simulink model "final_mppt_Algorithm_simuation_01"  (R2016a)
settings: Solver=VariableStepAuto  StartTime=0.0  StopTime=10.0  RelTol=1e-3
undefined symbols (not defined in the file or in its folder): sigbuilder_block
libraries: powerlib x12, simulink x2, powerlib_meascontrol x1
settings Model: Creator=Dell  LastModifiedBy=Dell

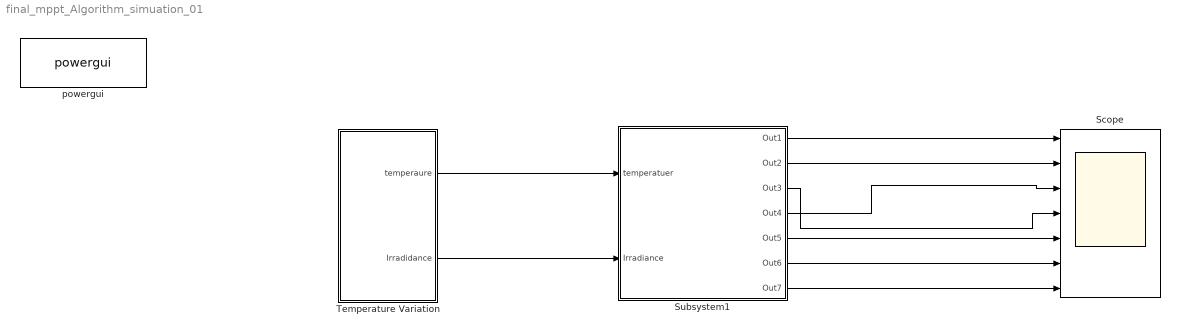
== system final_mppt_Algorithm_simuation_01 ==
  "Scope " : Scope  NumInputPorts=7
  Subsystem1 : Subsystem
  "Temperature Variation " : Subsystem  TreatAsAtomicUnit=on  VariantControl=Temperature
  powergui : powerlib/powergui  Priority=1  SimulationMode=Discrete  SolverType=Tustin  SampleTime=1e-6  frequency=60  SPID=off  DisableSnubberDevices=off  DisableRonSwitches=off  DisableVfSwitches=off  SwTol=0  DisplayEquations=off  Interpol=off  ExternalGateDelay=off  methode=off  Ts=0  FunctionMessages=off  echomessages=off  HookPort=off  EnableUseOfTLC=off  x0status=blocks  frequencyindice=0  Pbase=100e6  ErrMax=1e-4  Iterations=50  UnitsV=kV  UnitsW=MW  buscounter=0  RestoreLinks=warning  ResistiveCurrentMeasurement=off  Frange=[0:2:500]  Ylog=off  Xlog=on  ShowGrid=off  save=off  variable=ZData  structure=0  ZoomFFT=off  StartTime=0.0  cycles=1  DisplayStyle=1  fundamental=60  FreqAxis=off  MaxFrequency=1000  frequencyindicesteady=1  RmsSteady=1  display=off
  wires:
  "Temperature Variation "/1(temperaure) -> Subsystem1/1(temperatuer)
  "Temperature Variation "/2("Irradidance ") -> Subsystem1/2(Irradiance)
  Subsystem1/1(Out1) -> "Scope "/1
  Subsystem1/2(Out2) -> "Scope "/2
  Subsystem1/3(Out3) -> "Scope "/4
  Subsystem1/4(Out4) -> "Scope "/3
  Subsystem1/5(Out5) -> "Scope "/5
  Subsystem1/6(Out6) -> "Scope "/6
  Subsystem1/7(Out7) -> "Scope "/7

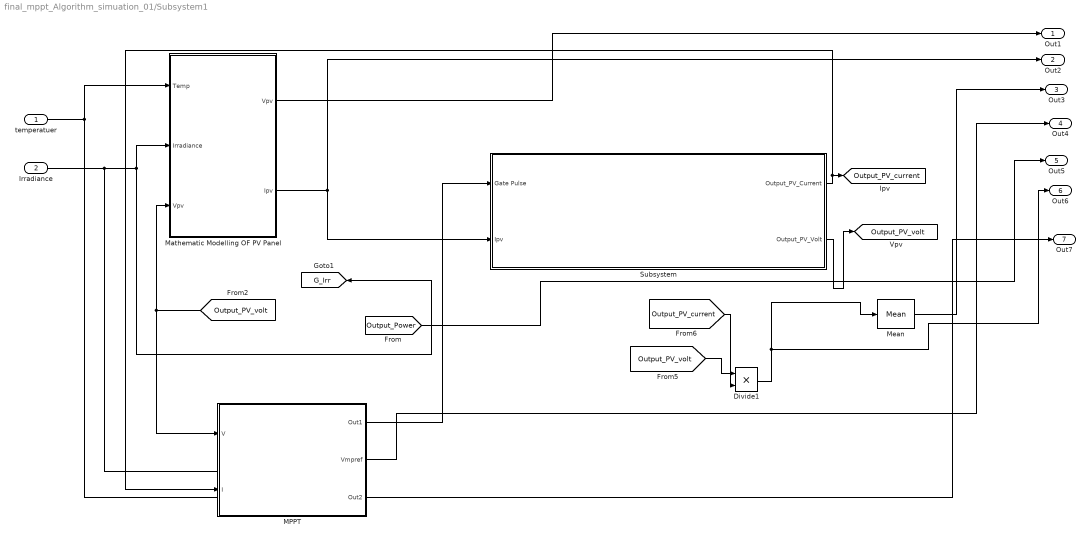
== system final_mppt_Algorithm_simuation_01/Subsystem1 ==
  temperatuer : Inport
  Irradiance : Inport  Port=2
  Divide1 : Product  Inputs=**
  MPPT : Subsystem
  Mathematic Modelling OF PV Panel : Subsystem
      mask Display:
      | plot([0.3 0.4],[0.4 0.8]);
      | plot([0.4 0.5],[0.4 0.8]);
      | plot([0.5 0.6],[0.4 0.8]);
      | plot([0.6 0.7],[0.4 0.8]);
      | plot([0.3 0.6],[0.4 0.4]);
      | plot([0.325 0.625],[0.5 0.5]);
      | plot([0.35 0.65],[0.6 0.6]);
      | plot([0.375 0.675],[0.7 0.7]);
      | plot([0.4 0.7],[0.8 0.8]);
      | text(0.52,0.75,'PV module (V)','horizontalAlignment', 'center');
  Mean : powerlib_meascontrol/Measurements/Mean  Freq=60  Vinit=0  Ts=0
  Subsystem : Subsystem
  Out1 : Outport
  Out2 : Outport  Port=2
  Out3 : Outport  Port=3
  Out4 : Outport  Port=4
  Out5 : Outport  Port=5
  Out6 : Outport  Port=6
  Out7 : Outport  Port=7
  tag scope: G_Irr=global, Output_PV_current=global, Output_PV_volt=global
  wires:
  [Output_PV_volt] -> Mathematic Modelling OF PV Panel/3(Vpv), MPPT/1(V)
  Irradiance/1 -> [G_Irr], Mathematic Modelling OF PV Panel/2(Irradiance)
  MPPT/2(Vmpref) -> Out4/1
  Mean/1 -> Out3/1
  Mathematic Modelling OF PV Panel/2(Ipv) -> Subsystem/2(Ipv), Out2/1
  MPPT/1(Out1) -> Subsystem/1(Gate Pulse)
  MPPT/3(Out2) -> Out7/1
  Mathematic Modelling OF PV Panel/1("Vpv ") -> Out1/1
  Divide1/1 -> Out6/1, Mean/1
  temperatuer/1 -> Mathematic Modelling OF PV Panel/1(Temp)
  Subsystem/1(Output_PV_Current) -> MPPT/2(I), [Output_PV_current]
  [Output_PV_volt] -> Divide1/1
  [Output_Power] -> Out5/1
  Subsystem/2(Output_PV_Volt) -> [Output_PV_volt]
  [Output_PV_current] -> Divide1/2

== system final_mppt_Algorithm_simuation_01/Temperature Variation  ==
  IRRADIANCE : Subsystem  Tag=STV Subsys  LoadFcn=sigbuilder_block('load');  StartFcn=sigbuilder_block('start');  StopFcn=sigbuilder_block('stop');  ClipboardFcn=sigbuilder_block('clipboard');  mask(Sigbuilder block){}
      mask help: Simulink:masks:SigbuilderBlock_MD
      mask init:
      | if ~strcmp(get_param(bdroot(gcbh),'SimulationStatus'),'stopped') tuvar = sigbuilder_block('maskInit'); end
      settings: CopyFcn=sigbuilder_block('copy');  DeleteFcn=sigbuilder_block('delete');  ModelCloseFcn=sigbuilder_block('modelClose');  PreSaveFcn=sigbuilder_block('preSave');  PauseFcn=sigbuilder_block('pause');  ContinueFcn=sigbuilder_block('continue');  NameChangeFcn=sigbuilder_block('namechange');  OpenFcn=sigbuilder_block('open',[6 28.2 1012.8 484.8 ]);  CloseFcn=sigbuilder_block('close');
      mask Display: plot(0, 0, 100, 100,[2, 2, 32, 32, 2], [68, 8, 8, 68, 68],[32, 2], [38, 38], [32, 19, 2],[53, 60, 44], [32, 17, 17, 2],[16, 16, 31, 31]);txt = getActiveGroup(gcbh);text(2, 100, txt,'verticalAlignment', 'top');
  TEMP : Subsystem  Tag=STV Subsys  LoadFcn=sigbuilder_block('load');  StartFcn=sigbuilder_block('start');  StopFcn=sigbuilder_block('stop');  ClipboardFcn=sigbuilder_block('clipboard');  mask(Sigbuilder block){}
      mask help: Simulink:masks:SigbuilderBlock_MD
      mask init:
      | if ~strcmp(get_param(bdroot(gcbh),'SimulationStatus'),'stopped') tuvar = sigbuilder_block('maskInit'); end
      settings: CopyFcn=sigbuilder_block('copy');  DeleteFcn=sigbuilder_block('delete');  ModelCloseFcn=sigbuilder_block('modelClose');  PreSaveFcn=sigbuilder_block('preSave');  PauseFcn=sigbuilder_block('pause');  ContinueFcn=sigbuilder_block('continue');  NameChangeFcn=sigbuilder_block('namechange');  OpenFcn=sigbuilder_block('open',[6 28.2 1012.8 484.8 ]);  CloseFcn=sigbuilder_block('close');
      mask Display: plot(0, 0, 100, 100,[2, 2, 32, 32, 2], [68, 8, 8, 68, 68],[32, 2], [38, 38], [32, 19, 2],[53, 60, 44], [32, 17, 17, 2],[16, 16, 31, 31]);txt = getActiveGroup(gcbh);text(2, 100, txt,'verticalAlignment', 'top');
  temperaure : Outport
  "Irradidance " : Outport  Port=2
  wires:
  TEMP/1(Signal 1) -> temperaure/1
  IRRADIANCE/1(Signal 2) -> "Irradidance "/1

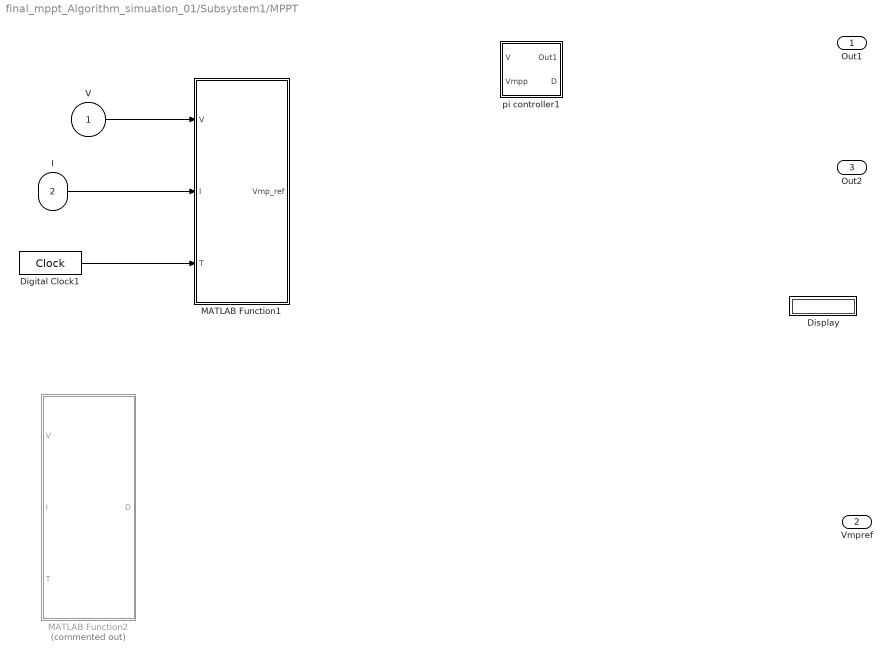
== system final_mppt_Algorithm_simuation_01/Subsystem1/MPPT ==
  V : Inport
  I : Inport  Port=2
  Digital Clock1 : DigitalClock  SampleTime=0.002
  Display : Display
  MATLAB Function1 : MATLAB Function  TreatAsAtomicUnit=on
  MATLAB Function2 : MATLAB Function  Commented=on  TreatAsAtomicUnit=on
  pi controller1 : Subsystem
  Out1 : Outport
  Vmpref : Outport  Port=2
  Out2 : Outport  Port=3
  wires:
  I/1 -> MATLAB Function1/2(I)
  V/1 -> MATLAB Function1/1(V)
  Digital Clock1/1 -> MATLAB Function1/3(T)

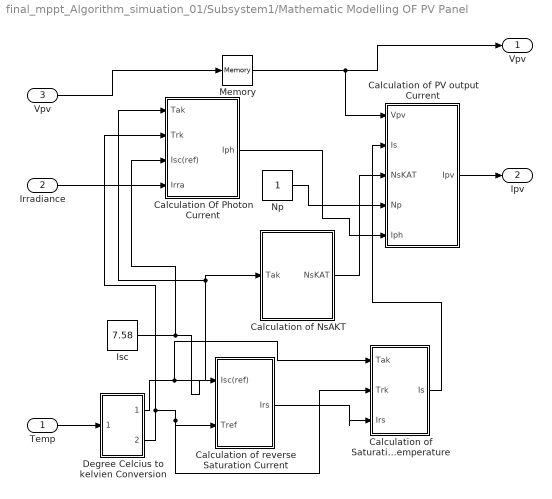
== system final_mppt_Algorithm_simuation_01/Subsystem1/Mathematic Modelling OF PV Panel ==
  Temp : Inport
  Irradiance : Inport  Port=2
  Vpv : Inport  Port=3
  "Calculation Of Photon Current " : Subsystem
  Calculation of Saturation Current Varies With Temperature : Subsystem
  Calculation of NsAKT : Subsystem
  "Calculation of PV output Current " : Subsystem
  Calculation of reverse Saturation Current : Subsystem
  Degree Celcius to kelvien Conversion : Subsystem
  Isc : Constant  Value=7.58
  Memory : Memory
  Np : Constant
  "Vpv " : Outport
  Ipv : Outport  Port=2
  wires:
  Calculation of Saturation Current Varies With Temperature/1(Is) -> "Calculation of PV output Current "/2(Is)
  Calculation of reverse Saturation Current/1(Irs) -> Calculation of Saturation Current Varies With Temperature/3("Irs ")
  Np/1 -> "Calculation of PV output Current "/4(Np)
  Temp/1 -> Degree Celcius to kelvien Conversion/1("Top ")
  "Calculation of PV output Current "/1("Ipv ") -> Ipv/1
  Irradiance/1 -> "Calculation Of Photon Current "/4(Irra)
  Degree Celcius to kelvien Conversion/1(Tak) -> Calculation of Saturation Current Varies With Temperature/1(Tak), "Calculation Of Photon Current "/1(Tak), Calculation of NsAKT/1("Tak ")
  "Calculation Of Photon Current "/1(Iph) -> "Calculation of PV output Current "/5(Iph)
  Calculation of NsAKT/1(NsKAT) -> "Calculation of PV output Current "/3(NsKAT)
  Isc/1 -> "Calculation Of Photon Current "/3(Isc(ref)), Calculation of reverse Saturation Current/1("Isc(ref) ")
  Degree Celcius to kelvien Conversion/2(Trk) -> "Calculation Of Photon Current "/2(Trk), Calculation of Saturation Current Varies With Temperature/2("Trk "), Calculation of reverse Saturation Current/2("Tref ")
  Vpv/1 -> Memory/1
  Memory/1 -> "Calculation of PV output Current "/1(Vpv), "Vpv "/1

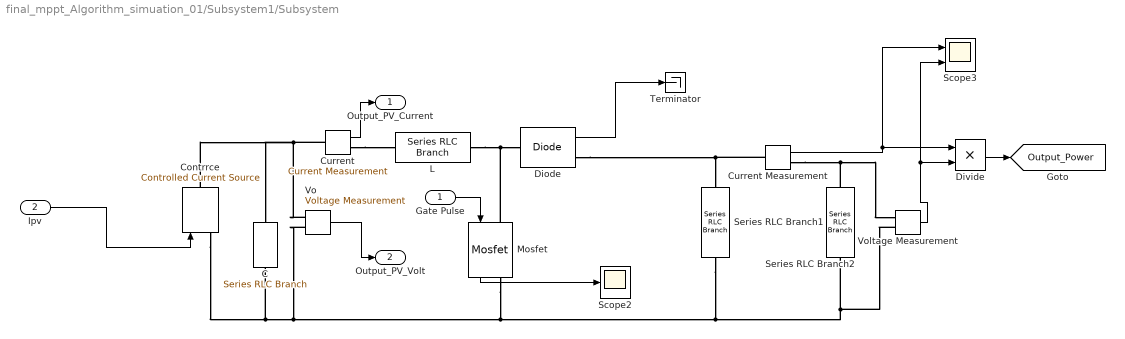
== system final_mppt_Algorithm_simuation_01/Subsystem1/Subsystem ==
  Gate Pulse : Inport
  Ipv : Inport  Port=2
  C : powerlib/Elements/Series RLC Branch  LConnTagsString=__new0  RConnTagsString=__new0  BranchType=C  Resistance=10  Inductance=5e-3  SetiL0=on  InitialCurrent=0  Capacitance=1e-6  Setx0=off  InitialVoltage=0  Measurements=None
  Contrrce : powerlib/Electrical Sources/Controlled Current Source  Initialize=on  Source_Type=DC  Amplitude=0  Phase=0  Frequency=0  Measurements=None
  "Current " : powerlib/Measurements/Current Measurement  PhasorSimulation=off  OutputType=Complex  PSBequivalent=0
  Current Measurement : powerlib/Measurements/Current Measurement  PhasorSimulation=off  OutputType=Complex  PSBequivalent=0
  Diode : powerlib/Power Electronics/Diode  Ron=0.001  Lon=0  Vf=0.8  IC=0  UseSnubber=off  Rs=500*0  Cs=250e-9*0  Measurements=on
  Divide : Product  Inputs=**
  L : powerlib/Elements/Series RLC Branch  LConnTagsString=__new0  RConnTagsString=__new0  BranchType=L  Resistance=10  Inductance=5e-3  SetiL0=on  InitialCurrent=0  Capacitance=1e-6  Setx0=off  InitialVoltage=0  Measurements=None
  Mosfet : powerlib/Power Electronics/Mosfet  Ron=0.1  Lon=0  Rd=0.01  Vfd=0  IC=0  Rs=1e5  Cs=inf  Measurements=on
  Scope2 : Scope
  Scope3 : Scope  NumInputPorts=2
  Series RLC Branch1 : powerlib/Elements/Series RLC Branch  LConnTagsString=__new0  RConnTagsString=__new0  BranchType=C  Resistance=1  Inductance=5e-3  SetiL0=on  InitialCurrent=0  Capacitance=270e-6  Setx0=on  InitialVoltage=0  Measurements=None
  Series RLC Branch2 : powerlib/Elements/Series RLC Branch  LConnTagsString=__new0  RConnTagsString=__new0  BranchType=R  Resistance=60  Inductance=5e-3  SetiL0=on  InitialCurrent=0  Capacitance=1e-6  Setx0=off  InitialVoltage=0  Measurements=None
  Terminator : Terminator
  Vo : powerlib/Measurements/Voltage Measurement  PhasorSimulation=off  OutputType=Complex  PSBequivalent=0
  Voltage Measurement : powerlib/Measurements/Voltage Measurement  PhasorSimulation=off  OutputType=Complex  PSBequivalent=0
  Output_PV_Current : Outport
  Output_PV_Volt : Outport  Port=2
  tag scope: Output_Power=global
  wires:
  Ipv/1 -> Contrrce/1
  Diode/1 -> Terminator/1
  Divide/1 -> [Output_Power]
  Voltage Measurement/1 -> Scope3/2, Divide/2
  Vo/1 -> Output_PV_Volt/1
  Gate Pulse/1 -> Mosfet/1
  "Current "/1 -> Output_PV_Current/1
  Current Measurement/1 -> Divide/1, Scope3/1
  Mosfet/1 -> Scope2/1
  connections:
  Diode/RConn1 -- Current Measurement/LConn1 -- Series RLC Branch1/LConn1
  Vo/LConn1 -- Contrrce/RConn1 -- C/LConn1 -- "Current "/LConn1
  Series RLC Branch2/LConn1 -- Current Measurement/RConn1 -- Voltage Measurement/LConn1
  Contrrce/LConn1 -- C/RConn1 -- Vo/LConn2 -- Mosfet/RConn1 -- Series RLC Branch1/RConn1 -- Voltage Measurement/LConn2 -- Series RLC Branch2/RConn1
  "Current "/RConn1 -- L/LConn1
  L/RConn1 -- Mosfet/LConn1 -- Diode/LConn1

== system final_mppt_Algorithm_simuation_01/Temperature Variation /IRRADIANCE ==
  Demux : Demux  Tag=STV Demux  Outputs=1
  FromWs : FromWorkspace  Tag=STV FromWs  VariableName=tuvar  SampleTime=0
      SigBuilderData=|
      | common.afterFinalStr = 'Extrapolate'
      | common.sampleTime = 0
      | dataSet.timeRange = [0 10]
      | dataSet.name = 'Group 1'
      | sbobj.Groups.Name = 'Group 1'
      | sbobj.Groups.Signals.Name = 'Signal 2'
      | sbobj.Groups.Signals.XData = [0 1 1 1.5 1.5 2 2 2.5 2.5 10]
      | sbobj.Groups.Signals.YData = [1 1 0.8 0.8 0.7 0.7 0.5 0.5 1 1]
  Signal 2 : Outport  Tag=STV Outport
  wires:
  FromWs/1 -> Demux/1
  Demux/1 -> Signal 2/1

== system final_mppt_Algorithm_simuation_01/Temperature Variation /TEMP ==
  Demux : Demux  Tag=STV Demux  Outputs=1
  FromWs : FromWorkspace  Tag=STV FromWs  VariableName=tuvar  SampleTime=0
      SigBuilderData=|
      | common.afterFinalStr = 'Extrapolate'
      | common.sampleTime = 0
      | dataSet.timeRange = [0 10]
      | dataSet.name = 'Group 1'
      | sbobj.Groups.Name = 'Group 1'
      | sbobj.Groups.Signals.Name = 'Signal 1'
      | sbobj.Groups.Signals.XData = [0 10]
      | sbobj.Groups.Signals.YData = [25 25]
  Signal 1 : Outport  Tag=STV Outport
  wires:
  Demux/1 -> Signal 1/1
  FromWs/1 -> Demux/1

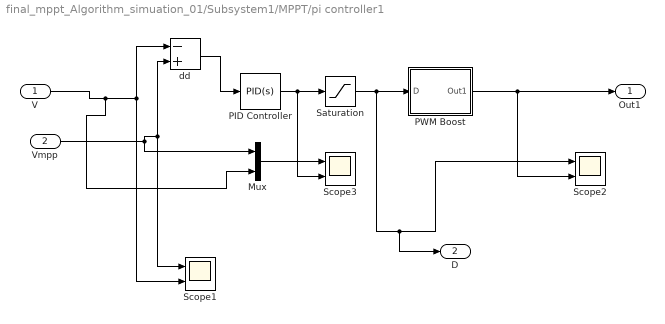
== system final_mppt_Algorithm_simuation_01/Subsystem1/MPPT/pi controller1 ==
  "V " : Inport
  Vmpp : Inport  Port=2
  Mux : Mux  Inputs=2
  PID Controller : simulink/Continuous/PID Controller  Controller=PID  TimeDomain=Continuous-time  SampleTime=-1  IntegratorMethod=Forward Euler  FilterMethod=Forward Euler  Form=Parallel  UseFilter=on  ControllerParametersSource=internal  P=0.2  I=10  D=0  N=100  InitialConditionSource=internal  InitialConditionForIntegrator=0  InitialConditionForFilter=0  ExternalReset=none  LimitOutput=off  UpperSaturationLimit=inf  LowerSaturationLimit=-inf  LinearizeAsGain=on  AntiWindupMode=none  Kb=1  TrackingMode=off  Kt=1  PParamMin=[]  PParamMax=[]  IParamMin=[]  IParamMax=[]  DParamMin=[]  DParamMax=[]  NParamMin=[]  NParamMax=[]  KbParamMin=[]  KbParamMax=[]  KtParamMin=[]  KtParamMax=[]  POutMin=[]  POutMax=[]  IOutMin=[]  IOutMax=[]  DOutMin=[]  DOutMax=[]  NOutMin=[]  NOutMax=[]  KbOutMin=[]  KbOutMax=[]  KtOutMin=[]  KtOutMax=[]  IntegratorOutMin=[]  IntegratorOutMax=[]  FilterOutMin=[]  FilterOutMax=[]  SumOutMin=[]  SumOutMax=[]  SumI1OutMin=[]  SumI1OutMax=[]  SumI2OutMin=[]  SumI2OutMax=[]  SumI3OutMin=[]  SumI3OutMax=[]  SumDOutMin=[]  SumDOutMax=[]  SaturationOutMin=[]  SaturationOutMax=[]  IntegratorContinuousStateAttributes=''  IntegratorStateMustResolveToSignalObject=off  IntegratorRTWStateStorageClass=Auto  FilterContinuousStateAttributes=''  FilterStateMustResolveToSignalObject=off  FilterRTWStateStorageClass=Auto  DifferentiatorICPrevScaledInput=0  DifferentiatorOutMin=[]  DifferentiatorOutMax=[]
  PWM Boost : Subsystem
  Saturation : Saturate  UpperLimit=0.85  LowerLimit=0.2
  Scope1 : Scope  NumInputPorts=2
  Scope2 : Scope  NumInputPorts=2
  Scope3 : Scope  NumInputPorts=2
  dd : Sum  Inputs=-+
  Out1 : Outport
  D : Outport  Port=2
  wires:
  "V "/1 -> Scope1/2, dd/1, Mux/2
  Mux/1 -> Scope3/1
  dd/1 -> PID Controller/1
  PID Controller/1 -> Saturation/1, Scope3/2
  Saturation/1 -> Scope2/1, D/1, PWM Boost/1(D)
  PWM Boost/1(Out1) -> Out1/1, Scope2/2
  Vmpp/1 -> Scope1/1, dd/2, Mux/1

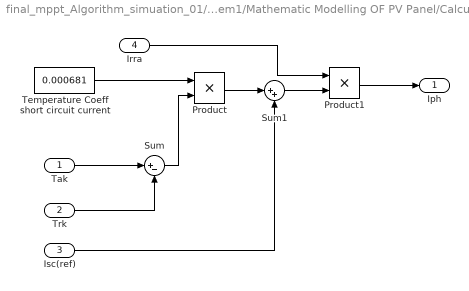
== system final_mppt_Algorithm_simuation_01/Subsystem1/Mathematic Modelling OF PV Panel/Calculation Of Photon Current  ==
  Tak : Inport
  Trk : Inport  Port=2
  Isc(ref) : Inport  Port=3
  Irra : Inport  Port=4
  Product : Product
  Product1 : Product
  Sum : Sum  Inputs=|+-
  Sum1 : Sum  Inputs=|++
  "Temperature Coeff short circuit current " : Constant  Value=0.000681
  Iph : Outport
  wires:
  Product/1 -> Sum1/1
  Trk/1 -> Sum/2
  "Temperature Coeff short circuit current "/1 -> Product/1
  Irra/1 -> Product1/1
  Isc(ref)/1 -> Sum1/2
  Tak/1 -> Sum/1
  Sum1/1 -> Product1/2
  Sum/1 -> Product/2
  Product1/1 -> Iph/1

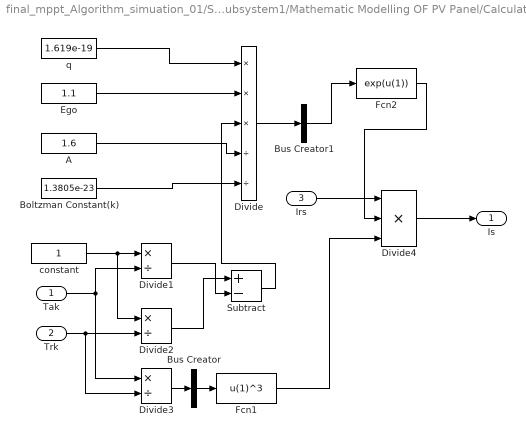
== system final_mppt_Algorithm_simuation_01/Subsystem1/Mathematic Modelling OF PV Panel/Calculation of Saturation Current Varies With Temperature ==
  Tak : Inport
  "Trk " : Inport  Port=2
  "Irs " : Inport  Port=3
  "A " : Constant  Value=1.6
  Boltzman Constant(k) : Constant  Value=1.3805e-23
  Bus Creator : BusCreator  Inputs=1
  Bus Creator1 : BusCreator  Inputs=1
  Divide : Product  Inputs=***//
  Divide1 : Product  Inputs=*/
  Divide2 : Product  Inputs=*/
  Divide3 : Product  Inputs=*/
  Divide4 : Product  Inputs=***
  Ego : Constant  Value=1.1
  Fcn1 : Fcn  Expr=u(1)^3
  Fcn2 : Fcn  Expr=exp(u(1))
  Subtract : Sum  Inputs=+-
  "constant " : Constant
  "q " : Constant  Value=1.619e-19
  Is : Outport
  wires:
  "constant "/1 -> Divide2/1, Divide1/1
  Bus Creator1/1 -> Fcn2/1
  Divide/1 -> Bus Creator1/1
  Divide1/1 -> Subtract/2
  Fcn1/1 -> Divide4/3
  Divide2/1 -> Subtract/1
  Tak/1 -> Divide1/2, Divide3/1
  Fcn2/1 -> Divide4/2
  "Trk "/1 -> Divide3/2, Divide2/2
  "A "/1 -> Divide/4
  Ego/1 -> Divide/2
  Subtract/1 -> Divide/3
  Boltzman Constant(k)/1 -> Divide/5
  "q "/1 -> Divide/1
  "Irs "/1 -> Divide4/1
  Divide4/1 -> Is/1
  Bus Creator/1 -> Fcn1/1
  Divide3/1 -> Bus Creator/1

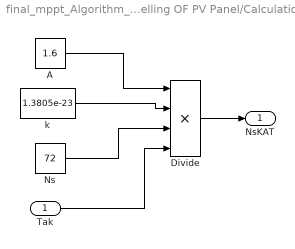
== system final_mppt_Algorithm_simuation_01/Subsystem1/Mathematic Modelling OF PV Panel/Calculation of NsAKT ==
  "Tak " : Inport
  A : Constant  Value=1.6
  Divide : Product  Inputs=****
  Ns : Constant  Value=72
  k : Constant  Value=1.3805e-23
  NsKAT : Outport
  wires:
  Ns/1 -> Divide/3
  A/1 -> Divide/1
  k/1 -> Divide/2
  "Tak "/1 -> Divide/4
  Divide/1 -> NsKAT/1

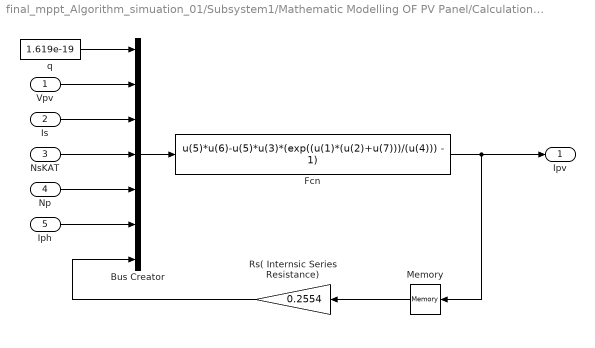
== system final_mppt_Algorithm_simuation_01/Subsystem1/Mathematic Modelling OF PV Panel/Calculation of PV output Current  ==
  Vpv : Inport
  Is : Inport  Port=2
  NsKAT : Inport  Port=3
  Np : Inport  Port=4
  Iph : Inport  Port=5
  Bus Creator : BusCreator  Inputs=7
  Fcn : Fcn  Expr=u(5)*u(6)-u(5)*u(3)*(exp((u(1)*(u(2)+u(7)))/(u(4))) - 1)
  Memory : Memory
  Rs( Internsic Series Resistance) : Gain  Gain=0.2554
  q : Constant  Value=1.619e-19
  "Ipv " : Outport
  wires:
  Vpv/1 -> Bus Creator/2
  Is/1 -> Bus Creator/3
  Fcn/1 -> Memory/1, "Ipv "/1
  Bus Creator/1 -> Fcn/1
  Rs( Internsic Series Resistance)/1 -> Bus Creator/7
  Iph/1 -> Bus Creator/6
  Np/1 -> Bus Creator/5
  q/1 -> Bus Creator/1
  NsKAT/1 -> Bus Creator/4
  Memory/1 -> Rs( Internsic Series Resistance)/1

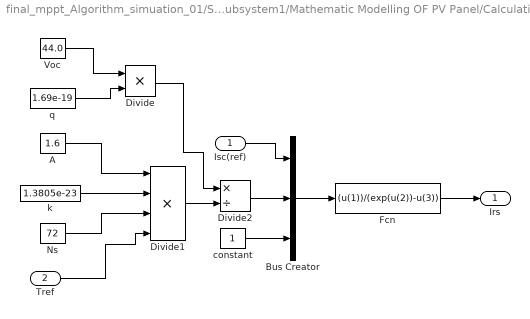
== system final_mppt_Algorithm_simuation_01/Subsystem1/Mathematic Modelling OF PV Panel/Calculation of reverse Saturation Current ==
  "Isc(ref) " : Inport
  "Tref " : Inport  Port=2
  A : Constant  Value=1.6
  Bus Creator : BusCreator  Inputs=3
  Divide : Product  Inputs=**
  Divide1 : Product  Inputs=****
  Divide2 : Product  Inputs=*/
  Fcn : Fcn  Expr=(u(1))/(exp(u(2))-u(3))
  Ns : Constant  Value=72
  Voc : Constant  Value=44.0
  "constant " : Constant
  k : Constant  Value=1.3805e-23
  q : Constant  Value=1.69e-19
  Irs : Outport
  wires:
  Voc/1 -> Divide/1
  Divide/1 -> Divide2/1
  k/1 -> Divide1/2
  "constant "/1 -> Bus Creator/3
  Divide2/1 -> Bus Creator/2
  Bus Creator/1 -> Fcn/1
  "Tref "/1 -> Divide1/4
  Fcn/1 -> Irs/1
  q/1 -> Divide/2
  A/1 -> Divide1/1
  "Isc(ref) "/1 -> Bus Creator/1
  Ns/1 -> Divide1/3
  Divide1/1 -> Divide2/2

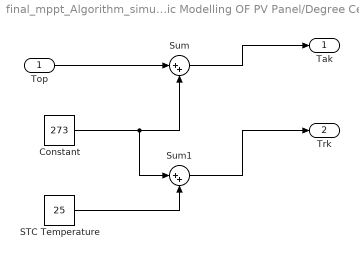
== system final_mppt_Algorithm_simuation_01/Subsystem1/Mathematic Modelling OF PV Panel/Degree Celcius to kelvien Conversion ==
  "Top " : Inport
  Constant : Constant  Value=273
  STC Temperature : Constant  Value=25
  Sum : Sum  Inputs=|++
  Sum1 : Sum  Inputs=|++
  Tak : Outport
  Trk : Outport  Port=2
  wires:
  Sum1/1 -> Trk/1
  Constant/1 -> Sum1/1, Sum/2
  "Top "/1 -> Sum/1
  Sum/1 -> Tak/1
  STC Temperature/1 -> Sum1/2

== system final_mppt_Algorithm_simuation_01/Subsystem1/MPPT/pi controller1/PWM Boost ==
  D : Inport
  Relational Operator : RelationalOperator  Operator=<=  OutDataTypeStr=boolean  ZeroCross=off
  Repeating Sequence : simulink/Sources/Repeating Sequence  rep_seq_t=[0 1/20000 1/10000]  rep_seq_y=[0 1 0]
  Scope : Scope  NumInputPorts=3
  Out1 : Outport
  wires:
  Repeating Sequence/1 -> Scope/1, Relational Operator/2
  Relational Operator/1 -> Out1/1, Scope/2
  D/1 -> Relational Operator/1, Scope/3

== matlab function final_mppt_Algorithm_simuation_01/Subsystem1/MPPT/MATLAB Function2 ==
  data: V input; D output; I input; T input
 function D = perturbandobserve(V,I,T)
persistent m1 p1 p2 v1;
persistent t1;
 if isempty(t1)
     t1=0;
     m1=0;
     p1=0;
     p2=0;
     v1=0;
end
i=I;v=V;
t=T;
step=0.1;
if t<=0.1
    m0=36;
    p1=v*i;
    t1=t
    m1=m0;
    v1=v;
    D=m1;
    return
end
if((t-t1)>0.1)
    p2=v*i;
    delp=p2-p1;
    delv=v-v1;
    if(delp==0)
        D=m1;
        p1=p2;
        t1=t;
        v1=v;
    return;  
    end
    
    if (delp>0)
        if (delv>0)
           m1=m1+step;
        else
           m1=m1-step;
        end
    else
        if (delv>0)
           m1=m1-step;
        else
           m1=m1+step;
        end
    end    
   D=m1;    
   p1=p2;
   t1=t;
   v1=v;
else
    D=m1;
end

 
 D=m1;
end

== matlab function final_mppt_Algorithm_simuation_01/Subsystem1/MPPT/MATLAB Function1 ==
  data: V input; Vmp_ref output; I input; T input
function Vmp_ref = perturbandobserve(V, I, T)

persistent V1 V0 V2 I1 I0 I2 P1 P0 P2 VmREF;

persistent t1;

dataType = 'double';

Voc=44;
i=I;
v=V;
t=T;
            if(t1)
                VmREF=0.8*Voc
                V0=0;
                V1=0;
                V2=0;
                I1=0;
                I2=0;
                I0=0;
                P1=0;
                P2=0;
                P0=0;
                t1=0;  
                Vmp_ref=VmREF;
                
                return;
            end
            
step=0.2*VmRef;

           
                
%             if()
% 
% 
%             end
% 
%             if()
% 
% 
% 
%             end

end
